simulink model "inverted_pendulum_template"  (R2021b)
settings: Solver=ode5  StartTime=0.0  StopTime=T  FixedStep=h  RelTol=1e-3  AbsTol=1e-6
undefined symbols (not defined in the file): h
settings Model: SimulationMode=external  ExtModeTrigDuration=12000  ExtModeTrigLevel=0.400000  Creator=jims  LastModifiedBy=lfalcone
settings SolverCC: AutoScaleAbsTol=off  AlgebraicLoopSolver=TrustRegion
settings DataIOCC: ExternalInput=[]  InitialState=[]  MaxDataPoints=5000  SaveFormat=Array  SignalLoggingSaveFormat=ModelDataLogs  SaveOutput=off  SaveTime=off  ReturnWorkspaceOutputs=off  SignalLoggingName=sigsOut
settings OptimizationCC: BooleanDataType=off  ExpressionDepthLimit=2147483647  InitFltsAndDblsToZero=on  LifeSpan=inf
settings DebuggingCC: SaveWithParameterizedLinksMsg=none  UnderspecifiedInitializationDetection=Classic  MergeDetectMultiDrivingBlocksExec=none  SignalResolutionControl=TryResolveAllWithWarning  MultiTaskDSMMsg=warning  MultiTaskCondExecSysMsg=none  IntegerOverflowMsg=none  FcnCallInpInsideContextMsg=warning  StateNameClashWarn=warning  SFUnexpectedBacktrackingDiag=warning  SFNoUnconditionalDefaultTransitionDiag=warning  SFExecutionAtInitializationDiag=none  IntegerSaturationMsg=none  ArithmeticOperatorsInVariantConditions=warning
settings HardwareCC: ProdBitPerPointer=32  ProdBitPerSizeT=32  ProdBitPerPtrDiffT=32  ProdLargestAtomicFloat=None  ProdIntDivRoundTo=Undefined  ProdEndianess=Unspecified  ProdWordSize=32  ProdHWDeviceType=32-bit Generic  TargetBitPerPointer=64  TargetBitPerSizeT=64  TargetBitPerPtrDiffT=64  TargetLongLongMode=on  TargetIntDivRoundTo=Zero  TargetEndianess=LittleEndian  TargetWordSize=64  TargetHWDeviceType=MATLAB Host  ProdEqTarget=off
settings ModelReferenceCC: PropagateSignalLabelsOutOfModel=off
settings SFSimCC: SimUseLocalCustomCode=off  CustomCodeUndefinedFunction=UseInterfaceOnly
settings RTWCC: SystemTargetFile=rtcon_pendulum_usb2.tlc  TemplateMakefile=rtcon_pendulum_vc_usb2_x64.tmf  RTWUseLocalCustomCode=off
settings CodeAppCC: StateflowObjectComments=on
settings STFCustomTargetCC: ModelReferenceCompliant=off  CombineOutputUpdateFcns=on  MatFileLogging=on  CPPClassGenCompliant=on  GRTInterface=off  SystemTargetFile=rtcon_pendulum_usb2.tlc
settings GRTTargetCC: TargetLangStandard=C89/C90 (ANSI)  ModelReferenceCompliant=off  ParMdlRefBuildCompliant=off  CompOptLevelCompliant=off  ConcurrentExecutionCompliant=off  UseToolchainInfoCompliant=off  ExtMode=on  ExtModeMexFile=rtcon_ext_comm
settings ConfigComp: CovMetricSettings=dw  CovSaveCumulativeToWorkspaceVar=on  CovSaveSingleToWorkspaceVar=on  CovExternalEMLEnable=off  CovSFcnEnable=off

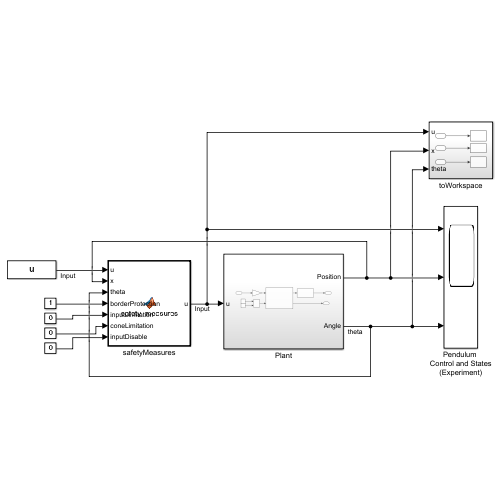
[thumbnail: Simulink's stored preview of the top-level diagram]
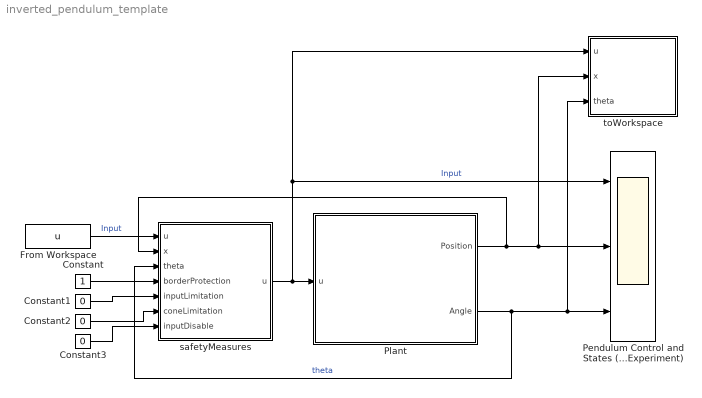
== system inverted_pendulum_template ==
  Constant : Constant
  Constant1 : Constant  Value=0
  Constant2 : Constant  Value=0
  Constant3 : Constant  Value=0
  From Workspace : FromWorkspace  VariableName=u
  Pendulum Control and States (Experiment) : Scope  NumInputPorts=3
  Plant : Subsystem
  safetyMeasures : MATLAB Function  TreatAsAtomicUnit=on
  toWorkspace : Subsystem
  wires:
  safetyMeasures/1(u) -> toWorkspace/1(u), Pendulum Control and States (Experiment)/1, Plant/1(u)  "Input"
  From Workspace/1 -> safetyMeasures/1("u ")  "Input"
  Constant/1 -> safetyMeasures/4(borderProtection)
  Constant1/1 -> safetyMeasures/5(inputLimitation)
  Constant2/1 -> safetyMeasures/6(coneLimitation)
  Plant/1(Position) -> safetyMeasures/2(x), toWorkspace/2(x), Pendulum Control and States (Experiment)/2
  Plant/2(Angle) -> safetyMeasures/3(theta), toWorkspace/3(theta), Pendulum Control and States (Experiment)/3  "theta"
  Constant3/1 -> safetyMeasures/7(inputDisable)

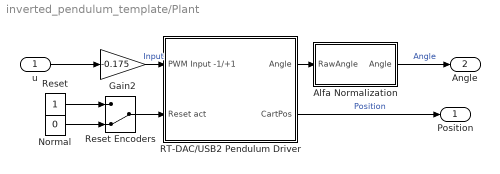
== system inverted_pendulum_template/Plant ==
  u : Inport
  Alfa Normalization : Subsystem  mask(Choose mode:){pos=Crane Controller}
      mask prompts: pos "Choose mode:"
      mask TypeOptions pos: Inverted Pendulum | Crane Controller
  Gain2 : Gain  Gain=-0.175
  Normal : Constant  Value=0
  "RT-DAC/USB2 Pendulum Driver " : Subsystem  mask{BoardID=-1, T0=h}
      mask prompts: BoardID "Board ID:"; T0 "Sample time:"
      mask help:
      | Serial number of the RT-DAC/USB2 board (BoardID). If only the single board is connected the Board ID should be -1.
      | Sanple time of the real-time executable.
      mask Display: image(imread('pendulum1.jpeg'))
  Reset : Constant
  Reset Encoders : ManualSwitch  CurrentSetting=0
  Position : Outport
  Angle : Outport  Port=2
  wires:
  "RT-DAC/USB2 Pendulum Driver "/1(Angle) -> Alfa Normalization/1(RawAngle)
  Normal/1 -> Reset Encoders/2
  Reset/1 -> Reset Encoders/1
  Alfa Normalization/1(Angle) -> Angle/1  "Angle"
  "RT-DAC/USB2 Pendulum Driver "/2(CartPos) -> Position/1  "Position"
  u/1 -> Gain2/1
  Reset Encoders/1 -> "RT-DAC/USB2 Pendulum Driver "/2(Reset act)
  Gain2/1 -> "RT-DAC/USB2 Pendulum Driver "/1(PWM Input -1/+1)  "Input"

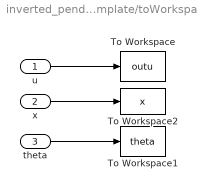
== system inverted_pendulum_template/toWorkspace ==
  u : Inport
  x : Inport  Port=2
  theta : Inport  Port=3
  To Workspace : ToWorkspace  VariableName=outu  SampleTime=-1
      settings: Save2DSignal=2-D array (concatenate along first dimension)
  To Workspace1 : ToWorkspace  VariableName=theta  SampleTime=-1
      settings: Save2DSignal=2-D array (concatenate along first dimension)
  To Workspace2 : ToWorkspace  VariableName=x  SampleTime=-1
      settings: Save2DSignal=2-D array (concatenate along first dimension)
  wires:
  u/1 -> To Workspace/1
  theta/1 -> To Workspace1/1
  x/1 -> To Workspace2/1

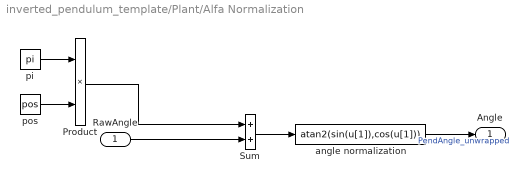
== system inverted_pendulum_template/Plant/Alfa Normalization ==
  RawAngle : Inport
  Product : Product  InputSameDT=on  SaturateOnIntegerOverflow=on  OutDataTypeStr=Inherit: Same as first input
  Sum : Sum  InputSameDT=on  SaturateOnIntegerOverflow=on  OutDataTypeStr=Inherit: Same as first input
  angle normalization : Fcn  Expr=atan2(sin(u[1]),cos(u[1]))
  pi : Constant  Value=pi
  pos : Constant  Value=pos
  Angle : Outport  InitialOutput=0  VectorParamsAs1DForOutWhenUnconnected=off
  wires:
  angle normalization/1 -> Angle/1  "PendAngle_unwrapped"
  Sum/1 -> angle normalization/1
  RawAngle/1 -> Sum/2
  pi/1 -> Product/1
  pos/1 -> Product/2
  Product/1 -> Sum/1

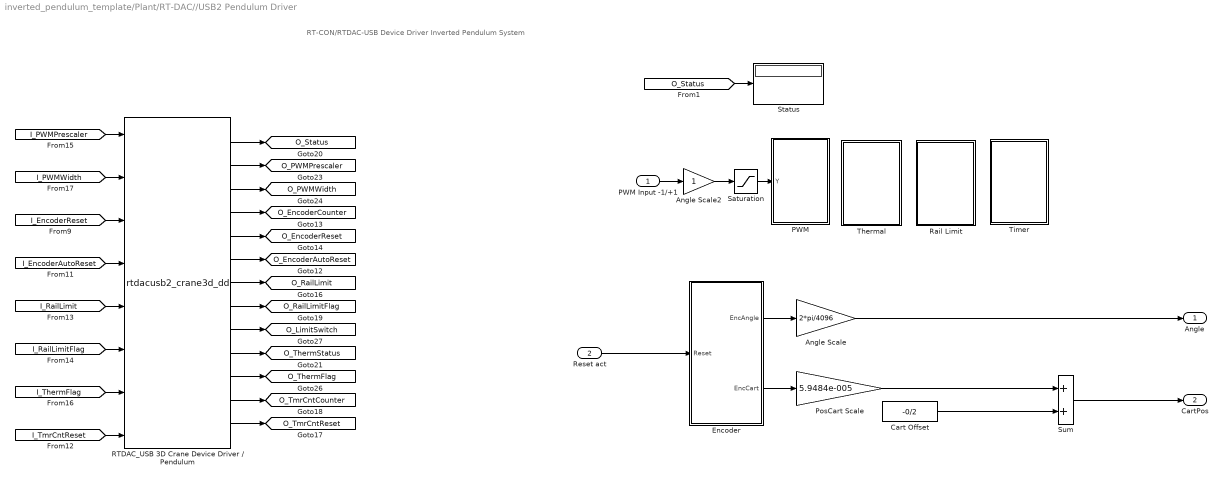
== system inverted_pendulum_template/Plant/RT-DAC//USB2 Pendulum Driver  ==
  note: RT-CON/RTDAC-USB Device Driver
      | Inverted Pendulum System
  PWM Input -1/+1 : Inport
  Reset act : Inport  Port=2
  Angle Scale : Gain  Gain=2*pi/4096  OutDataTypeStr=Inherit: Same as input  ParamDataTypeStr=Inherit: Same as input
  Angle Scale2 : Gain  OutDataTypeStr=Inherit: Same as input  ParamDataTypeStr=Inherit: Same as input
  Cart Offset : Constant  Value=-0/2
  Encoder : Subsystem
  PWM : Subsystem
      mask Display: disp('PWM')
  PosCart Scale : Gain  Gain=5.9484e-005  OutDataTypeStr=Inherit: Same as input  ParamDataTypeStr=Inherit: Same as input
  RTDAC_USB 3D Crane Device Driver / Pendulum : S-Function  FunctionName=rtdacusb2_crane3d_dd  Parameters=-1, 0.01  SFunctionDeploymentMode=off  EnableBusSupport=off
  Rail Limit : Subsystem
      mask Display: disp('Rail\nLimit')
  Saturation : Saturate  UpperLimit=1  LowerLimit=-1
  Status : Display
      settings: Format=hex (Stored Integer)
  Sum : Sum  InputSameDT=on  SaturateOnIntegerOverflow=on  OutDataTypeStr=Inherit: Same as first input
  Thermal : Subsystem
      mask Display: disp('Thermal')
  Timer : Subsystem
      mask Display: disp('Timer')
  Angle : Outport  VectorParamsAs1DForOutWhenUnconnected=off
  CartPos : Outport  Port=2  VectorParamsAs1DForOutWhenUnconnected=off
  tag scope: O_EncoderAutoReset=global, O_EncoderCounter=global, O_EncoderReset=global, O_LimitSwitch=global, O_PWMPrescaler=global, O_PWMWidth=global, O_RailLimit=global, O_RailLimitFlag=global, O_Status=global, O_ThermFlag=global, O_ThermStatus=global, O_TmrCntCounter=global, O_TmrCntReset=global
  wires:
  RTDAC_USB 3D Crane Device Driver / Pendulum/4 -> [O_EncoderCounter]
  [I_EncoderAutoReset] -> RTDAC_USB 3D Crane Device Driver / Pendulum/4
  RTDAC_USB 3D Crane Device Driver / Pendulum/7 -> [O_RailLimit]
  [I_RailLimit] -> RTDAC_USB 3D Crane Device Driver / Pendulum/5
  RTDAC_USB 3D Crane Device Driver / Pendulum/6 -> [O_EncoderAutoReset]
  [I_RailLimitFlag] -> RTDAC_USB 3D Crane Device Driver / Pendulum/6
  RTDAC_USB 3D Crane Device Driver / Pendulum/10 -> [O_ThermStatus]
  RTDAC_USB 3D Crane Device Driver / Pendulum/5 -> [O_EncoderReset]
  RTDAC_USB 3D Crane Device Driver / Pendulum/9 -> [O_LimitSwitch]
  [I_EncoderReset] -> RTDAC_USB 3D Crane Device Driver / Pendulum/3
  RTDAC_USB 3D Crane Device Driver / Pendulum/8 -> [O_RailLimitFlag]
  [I_TmrCntReset] -> RTDAC_USB 3D Crane Device Driver / Pendulum/8
  RTDAC_USB 3D Crane Device Driver / Pendulum/3 -> [O_PWMWidth]
  RTDAC_USB 3D Crane Device Driver / Pendulum/13 -> [O_TmrCntReset]
  RTDAC_USB 3D Crane Device Driver / Pendulum/11 -> [O_ThermFlag]
  [I_PWMWidth] -> RTDAC_USB 3D Crane Device Driver / Pendulum/2
  [I_ThermFlag] -> RTDAC_USB 3D Crane Device Driver / Pendulum/7
  [I_PWMPrescaler] -> RTDAC_USB 3D Crane Device Driver / Pendulum/1
  RTDAC_USB 3D Crane Device Driver / Pendulum/1 -> [O_Status]
  RTDAC_USB 3D Crane Device Driver / Pendulum/2 -> [O_PWMPrescaler]
  RTDAC_USB 3D Crane Device Driver / Pendulum/12 -> [O_TmrCntCounter]
  [O_Status] -> Status/1
  PWM Input -1/+1/1 -> Angle Scale2/1
  Reset act/1 -> Encoder/1(Reset)
  Cart Offset/1 -> Sum/2
  Sum/1 -> CartPos/1
  PosCart Scale/1 -> Sum/1
  Saturation/1 -> PWM/1(Y)
  Encoder/2(EncCart) -> PosCart Scale/1
  Encoder/1(EncAngle) -> Angle Scale/1
  Angle Scale2/1 -> Saturation/1
  Angle Scale/1 -> Angle/1

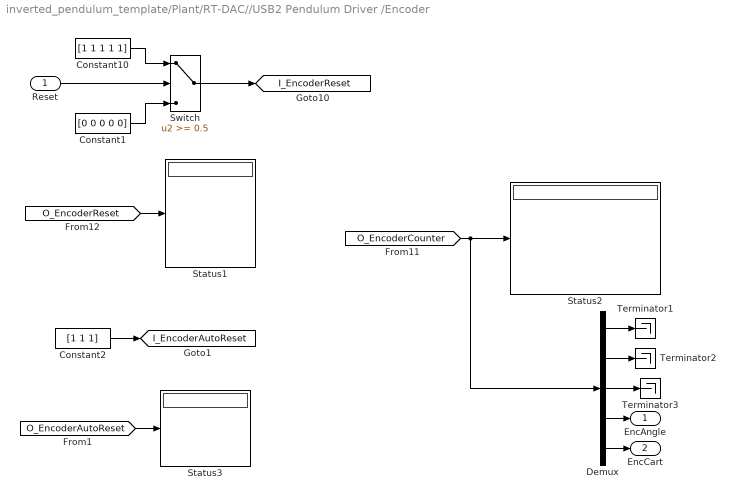
== system inverted_pendulum_template/Plant/RT-DAC//USB2 Pendulum Driver /Encoder ==
  Reset : Inport
  Constant1 : Constant  Value=[0 0 0 0 0]
  Constant10 : Constant  Value=[1 1 1 1 1]
  Constant2 : Constant  Value=[1 1 1]
  Demux : Demux  Outputs=5
  Status1 : Display
  Status2 : Display
  Status3 : Display
  Switch : Switch  Threshold=0.5  InputSameDT=on
  Terminator1 : Terminator
  Terminator2 : Terminator
  Terminator3 : Terminator
  EncAngle : Outport  VectorParamsAs1DForOutWhenUnconnected=off
  EncCart : Outport  Port=2  VectorParamsAs1DForOutWhenUnconnected=off
  tag scope: I_EncoderAutoReset=global, I_EncoderReset=global
  wires:
  [O_EncoderAutoReset] -> Status3/1
  Constant2/1 -> [I_EncoderAutoReset]
  Demux/5 -> EncCart/1
  Demux/4 -> EncAngle/1
  Constant1/1 -> Switch/3
  Constant10/1 -> Switch/1
  Switch/1 -> [I_EncoderReset]
  Reset/1 -> Switch/2
  Demux/3 -> Terminator3/1
  Demux/2 -> Terminator2/1
  Demux/1 -> Terminator1/1
  [O_EncoderCounter] -> Status2/1, Demux/1
  [O_EncoderReset] -> Status1/1

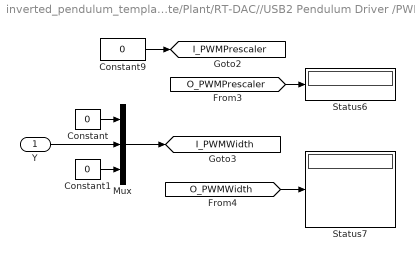
== system inverted_pendulum_template/Plant/RT-DAC//USB2 Pendulum Driver /PWM ==
  Y : Inport
  Constant : Constant  Value=0
  Constant1 : Constant  Value=0
  Constant9 : Constant  Value=0
  Mux : Mux  Inputs=3
  Status6 : Display
  Status7 : Display
  tag scope: I_PWMPrescaler=global, I_PWMWidth=global
  wires:
  Constant1/1 -> Mux/3
  Mux/1 -> [I_PWMWidth]
  Y/1 -> Mux/2
  Constant/1 -> Mux/1
  Constant9/1 -> [I_PWMPrescaler]
  [O_PWMPrescaler] -> Status6/1
  [O_PWMWidth] -> Status7/1

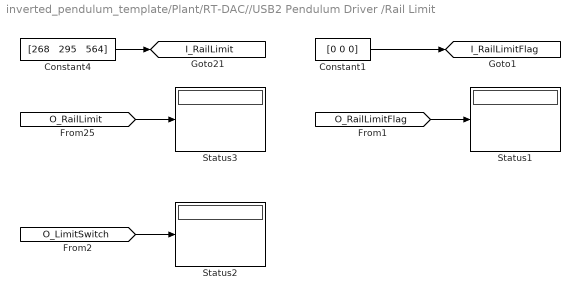
== system inverted_pendulum_template/Plant/RT-DAC//USB2 Pendulum Driver /Rail Limit ==
  Constant1 : Constant  Value=[0 0 0]
  Constant4 : Constant  Value="[268   295   564]"
  Status1 : Display
  Status2 : Display
  Status3 : Display
  tag scope: I_RailLimit=global, I_RailLimitFlag=global
  wires:
  [O_LimitSwitch] -> Status2/1
  Constant1/1 -> [I_RailLimitFlag]
  [O_RailLimitFlag] -> Status1/1
  Constant4/1 -> [I_RailLimit]
  [O_RailLimit] -> Status3/1

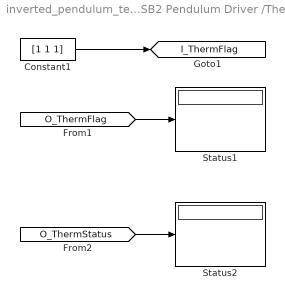
== system inverted_pendulum_template/Plant/RT-DAC//USB2 Pendulum Driver /Thermal ==
  Constant1 : Constant  Value=[1 1 1]
  Status1 : Display
  Status2 : Display
  tag scope: I_ThermFlag=global
  wires:
  [O_ThermFlag] -> Status1/1
  Constant1/1 -> [I_ThermFlag]
  [O_ThermStatus] -> Status2/1

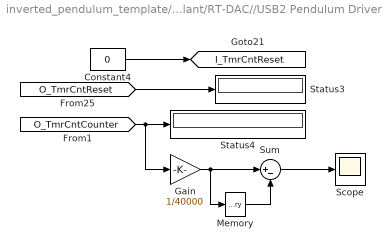
== system inverted_pendulum_template/Plant/RT-DAC//USB2 Pendulum Driver /Timer ==
  Constant4 : Constant  Value=0
  Gain : Gain  Gain=1/40000  SaturateOnIntegerOverflow=on  OutDataTypeStr=Inherit: Same as input  ParamDataTypeStr=Inherit: Same as input
  Memory : Memory
  Scope : Scope
  Status3 : Display
  Status4 : Display
  Sum : Sum  Inputs=|+-  InputSameDT=on  SaturateOnIntegerOverflow=on  OutDataTypeStr=Inherit: Same as first input
  tag scope: I_TmrCntReset=global
  wires:
  Sum/1 -> Scope/1
  Memory/1 -> Sum/2
  Gain/1 -> Memory/1, Sum/1
  [O_TmrCntCounter] -> Gain/1, Status4/1
  [O_TmrCntReset] -> Status3/1
  Constant4/1 -> [I_TmrCntReset]

== matlab function inverted_pendulum_template/safetyMeasures ==
  data: u input; u output; x input; theta input; borderProtection input; inputLimitation input; coneLimitation input; inputDisable input
function u = safety_measures(u, x, theta, borderProtection, inputLimitation, coneLimitation, inputDisable)

% border protection parameters
forceFieldStrenght = 1;
leftborder = 1;
rightborder = -1;
safety_margin = 0.30;

% input limitation parameters
inputLimit = 1.5;

% cone limitation parameters
coneWidth = 35; % deg

% execution
if inputLimitation
    if u > inputLimit
        u = inputLimit;
    elseif u < -inputLimit
        u = -inputLimit;
    end
end

if coneLimitation
    if abs(theta) > coneWidth/180*pi
        u = 0;
    end
end

if borderProtection 
    if(x < rightborder + safety_margin)
        u = forceFieldStrenght;
    end
    if(x > leftborder - safety_margin)
        u = -forceFieldStrenght;
    end
end

if inputDisable
    u = 0;
end

end
